simulink model "Disturbance"  (R2015a)
settings: Solver=ode1  StartTime=0.0  StopTime=5  FixedStep=0.0001  RelTol=1e-3
PostLoadFcn:
  | , if any(exist('dsrtsu_mdlpostloadfcn', 'file') == [2, 3, 6]), try dsrtsu_mdlpostloadfcn('Execute', bdroot); catch fprintf('Error in PostLoadFcn (dsrtsu_mdlpostloadfcn) for model "%s":\n %s\n', bdroot, lasterr); end, end,
libraries: simulink_extras x1
settings Model: DSRTSU_INTERNAL_RTI_VER=450  DSRTSU_INTERNAL_RTI_TYPE=rti1006  DSRTSU_INTERNAL_RTIFPGA=40  Creator=NSEE  LastModifiedBy=NSEE
settings OptimizationCC: BlockReduction=off  OptimizeBlockIOStorage=off  BufferReuse=off  GlobalBufferReuse=off  ExpressionFolding=off  LocalBlockOutputs=off
settings HardwareCC: ProdIntDivRoundTo=Zero  ProdEndianess=LittleEndian  ProdHWDeviceType=Generic->Custom  TargetIntDivRoundTo=Zero  TargetEndianess=LittleEndian  TargetHWDeviceType=Generic->Custom
settings RTWCC: SystemTargetFile=rti1006.tlc  MakeCommand=make_rti  TemplateMakefile=rti1006.tmf  Description=dSPACE DS1006 Hardware Platform
settings STFCustomTargetCC: GenerateSampleERTMain=off  ParMdlRefBuildCompliant=on  GeneratePreprocessorConditionals=Disable all  ERTCustomFileBanners=off  MatFileLogging=on  SupportNonInlinedSFcns=on  SupportVariableSizeSignals=off  MATLABClassNameForMDSCustomization=Simulink.SoftwareTarget.GRTCustomization  GRTInterface=on  SystemTargetFile=rti1006.tlc
settings GRTTargetCC: CompOptLevelCompliant=off  ConcurrentExecutionCompliant=off  CombineOutputUpdateFcns=off  CPPClassGenCompliant=off  GRTInterface=on  ExtModeMexFile=noextcomm

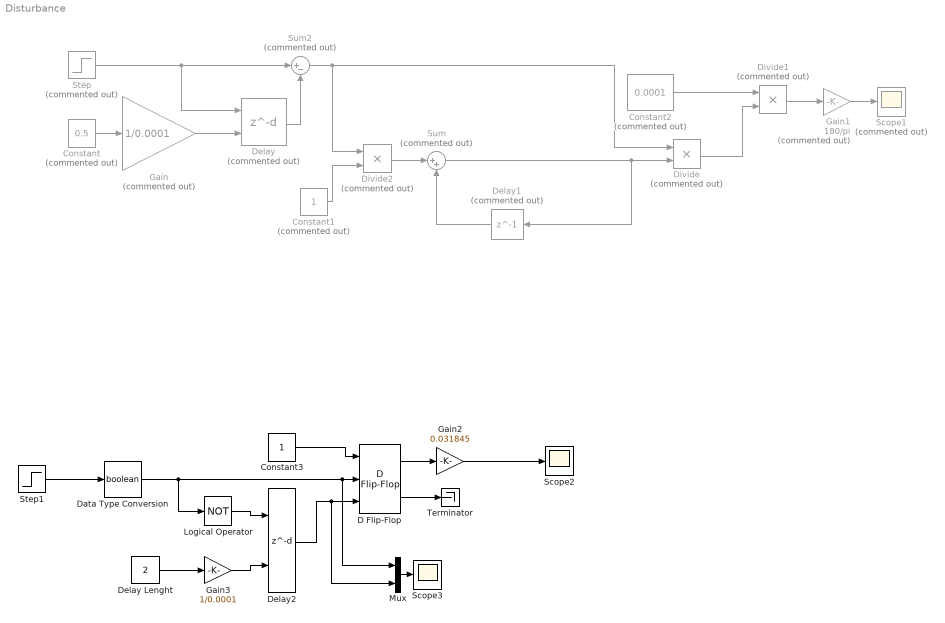
== system Disturbance ==
  Constant : Constant  Commented=on  Value=0.5
  Constant1 : Constant  Commented=on
  Constant2 : Constant  Commented=on  Value=0.0001
  Constant3 : Constant  OutDataTypeStr=boolean
  D Flip-Flop : simulink_extras/Flip Flops/D Flip-Flop
  Data Type Conversion : DataTypeConversion  OutDataTypeStr=boolean
  Delay : Delay  Commented=on  DelayLengthSource=Input port  DelayLength=1/0.001  DelayLengthUpperLimit=100000  InitialCondition=0
      settings: InputPortMap=u0,p1
  Delay Lenght : Constant  Value=2  OutDataTypeStr=double
  Delay1 : Delay  Commented=on  DelayLength=1  InitialCondition=0
  Delay2 : Delay  DelayLengthSource=Input port  DelayLengthUpperLimit=100000  InitialCondition=1
      settings: InputPortMap=u0,p1
  Divide : Product  Commented=on  Inputs=**
  Divide1 : Product  Commented=on  Inputs=**
  Divide2 : Product  Commented=on  Inputs=**
  Gain : Gain  Commented=on  Gain=1/0.0001
  Gain1 : Gain  Commented=on  Gain=180/pi
  Gain2 : Gain  Gain=0.031845  ParamDataTypeStr=double
  Gain3 : Gain  Gain=1/0.0001
  Logical Operator : Logic  Operator=NOT  AllPortsSameDT=off  OutDataTypeStr=boolean
  Mux : Mux  Inputs=2
  Scope1 : Scope  Commented=on
      settings: YMin=0  YMax=30
  Scope2 : Scope
      settings: YMin=0  YMax=0.0325
  Scope3 : Scope
      settings: TimeRange=10  SaveName=ScopeData3
  Step : Step  Commented=on  SampleTime=0
  Step1 : Step  SampleTime=0
  Sum : Sum  Commented=on  Inputs=|++
  Sum2 : Sum  Commented=on  Inputs=|+-
  Terminator : Terminator
  wires:
  Sum/1 -> Divide/2, Delay1/1
  Sum2/1 -> Divide2/1, Divide/1
  Delay1/1 -> Sum/2
  Step/1 -> Delay/1, Sum2/1
  Delay/1 -> Sum2/2
  Gain/1 -> Delay/2
  Constant/1 -> Gain/1
  Divide/1 -> Divide1/2
  Constant2/1 -> Divide1/1
  Divide1/1 -> Gain1/1
  Gain1/1 -> Scope1/1
  Constant1/1 -> Divide2/2
  Divide2/1 -> Sum/1
  Constant3/1 -> D Flip-Flop/1
  Delay2/1 -> Mux/2, D Flip-Flop/3
  Logical Operator/1 -> Delay2/1
  Step1/1 -> Data Type Conversion/1
  D Flip-Flop/1 -> Gain2/1
  Gain2/1 -> Scope2/1
  D Flip-Flop/2 -> Terminator/1
  Delay Lenght/1 -> Gain3/1
  Mux/1 -> Scope3/1
  Gain3/1 -> Delay2/2
  Data Type Conversion/1 -> Logical Operator/1, Mux/1, D Flip-Flop/2
